simulink model "Robot_DH"  (R2023b)
settings: Solver=VariableStepAuto  StartTime=0.0  StopTime=7  RelTol=1e-3
values from neighbouring files (symbols this model uses):
  a1 = 40    [FK.m]    (also in IK_Analytical.m = 0.04; IK_MDH.m = 0.04; IK_Position.m = 0.04; IK_Solver.m = 0.04)
  a2 = 275    [FK.m]    (also in IK_Analytical.m = 0.275; IK_MDH.m = 0.275; IK_Position.m = 0.275; IK_Solver.m = 0.275)
  a3 = 25    [FK.m]    (also in IK_Analytical.m = 0.025; IK_MDH.m = 0.025; IK_Position.m = 0.025; IK_Solver.m = 0.025)
  d1 = 342    [FK.m]    (also in IK_Analytical.m = 0.342; IK_MDH.m = 0.342; IK_Position.m = 0.342; IK_Solver.m = 0.342)
  d4 = 280    [FK.m]    (also in IK_Analytical.m = 0.28; IK_MDH.m = 0.28; IK_Position.m = 0.28; IK_Solver.m = 0.28)
  DH = @(a,alpha,d,theta) [      cos(theta)            -sin(theta)             0              a ... (first row only)    [FK.m]    (also in set_mode_parameter.m = [)
  dt = 73    [FK.m]    (also in IK_Position.m = 0.073; IK_Solver.m = 0.073; diagnose_IK.m = 0.073; init_robot_arm_system.m = 0.087)
  fc1 = 0    [set_mode_parameter.m]
  fc2 = 0    [set_mode_parameter.m]
  fc3 = 0    [set_mode_parameter.m]
  fc4 = 0    [set_mode_parameter.m]
  fc5 = 0    [set_mode_parameter.m]
  fc6 = 0    [set_mode_parameter.m]
  fv1 = 0    [set_mode_parameter.m]
  fv2 = 0    [set_mode_parameter.m]
  fv3 = 0    [set_mode_parameter.m]
  fv4 = 0    [set_mode_parameter.m]
  fv5 = 0    [set_mode_parameter.m]
  fv6 = 0    [set_mode_parameter.m]
  Ia1 = 0    [set_mode_parameter.m]
  Ia2 = 0    [set_mode_parameter.m]
  Ia3 = 0    [set_mode_parameter.m]
  Ia4 = 0    [set_mode_parameter.m]
  Ia5 = 0    [set_mode_parameter.m]
  Ia6 = 0    [set_mode_parameter.m]
  Ic111 = 0    [set_mode_parameter.m]
  Ic112 = 0    [set_mode_parameter.m]
  Ic113 = 0    [set_mode_parameter.m]
  Ic122 = 0    [set_mode_parameter.m]
  Ic123 = 0    [set_mode_parameter.m]
  Ic133 = 1.3676    [set_mode_parameter.m]
  Ic211 = 8.8194    [set_mode_parameter.m]
  Ic212 = 0    [set_mode_parameter.m]
  Ic213 = 0    [set_mode_parameter.m]
  Ic222 = 6.0549    [set_mode_parameter.m]
  Ic223 = 0    [set_mode_parameter.m]
  Ic233 = 0.9569    [set_mode_parameter.m]
  Ic311 = 0.0332    [set_mode_parameter.m]
  Ic312 = 0    [set_mode_parameter.m]
  Ic313 = 0    [set_mode_parameter.m]
  Ic322 = 1.8442    [set_mode_parameter.m]
  Ic323 = 0    [set_mode_parameter.m]
  Ic333 = 1.0560    (= 1.056)    [set_mode_parameter.m]
  Ic411 = 0.1448    [set_mode_parameter.m]
  Ic412 = 0    [set_mode_parameter.m]
  Ic413 = 0    [set_mode_parameter.m]
  Ic422 = 0.0015    [set_mode_parameter.m]
  Ic423 = 0    [set_mode_parameter.m]
  Ic433 = 0.0822    [set_mode_parameter.m]
  Ic511 = 0    [set_mode_parameter.m]
  Ic512 = 0    [set_mode_parameter.m]
  Ic513 = 0    [set_mode_parameter.m]
  Ic522 = 0.0121    [set_mode_parameter.m]
  Ic523 = 0    [set_mode_parameter.m]
  Ic533 = 0.0299    [set_mode_parameter.m]
  Ic611 = 0.0134    [set_mode_parameter.m]
  Ic612 = 0    [set_mode_parameter.m]
  Ic613 = 0    [set_mode_parameter.m]
  Ic622 = 0    [set_mode_parameter.m]
  Ic623 = 0    [set_mode_parameter.m]
  Ic633 = 0.0051    [set_mode_parameter.m]
  joint_limits = joint_limits_deg    [set_mode_parameter.m]
  m = (c1*px + s1*py) - dt*(c1*ax + s1*ay) - a1    [IK_6DOF_Robot.m]    (also in IK_MDH.m = pwx_1 - a1; IK_MDH_Robot.m = rho - a1)
  m1 = 0.167    [set_mode_parameter.m]
  m2 = 1    [set_mode_parameter.m]
  m3 = 0.5    [set_mode_parameter.m]
  m4 = 0.333    [set_mode_parameter.m]
  m5 = 0.25    [set_mode_parameter.m]
  m6 = 0.2    [set_mode_parameter.m]
  mc11 = 0    [set_mode_parameter.m]
  mc12 = 0    [set_mode_parameter.m]
  mc13 = 0.2    [set_mode_parameter.m]
  mc21 = 0.1291    [set_mode_parameter.m]
  mc22 = 0    [set_mode_parameter.m]
  mc23 = 3.3117    [set_mode_parameter.m]
  mc31 = 1.6484    [set_mode_parameter.m]
  mc32 = 0    [set_mode_parameter.m]
  mc33 = 0.8748    [set_mode_parameter.m]
  mc41 = 0.3200    (= 0.32)    [set_mode_parameter.m]
  mc42 = 0.2324    [set_mode_parameter.m]
  mc43 = 0.7083    [set_mode_parameter.m]
  mc51 = 0.4574    [set_mode_parameter.m]
  mc52 = 0    [set_mode_parameter.m]
  mc53 = 0.6427    [set_mode_parameter.m]
  mc61 = 0.3200    (= 0.32)    [set_mode_parameter.m]
  mc62 = -0.0513    [set_mode_parameter.m]
  mc63 = 0.6417    [set_mode_parameter.m]
  MDH = [ ... (first row only)    [FK_MDH.m]    (also in optimize_MDH_params.m = [x(1:6), [0; 0; 0.275; 0.025; 0; 0],         [0.342; 0.040; ; set_mode_parameter.m; test_222.m)
  N = size(waypoints, 2)    [run_trajectory.m]
  R1 = [0 0 1 ... (first row only)    [set_mode_parameter.m]    (also in test_20251215.m)
  s = zc - d(1)    [inverse_kinematics_6dof.m]
  XB4 = SerialLink([L1 L2 L3 L4 L5 L6], 'name', 'XB4')    [Toolbox_Motheds_1.m]
undefined symbols (not defined in the file or in its folder): X, Y, Z
libraries: sm_lib x56, nesl_utility x31, robotcorelib x2, simulink x2
(part 2 of 2)

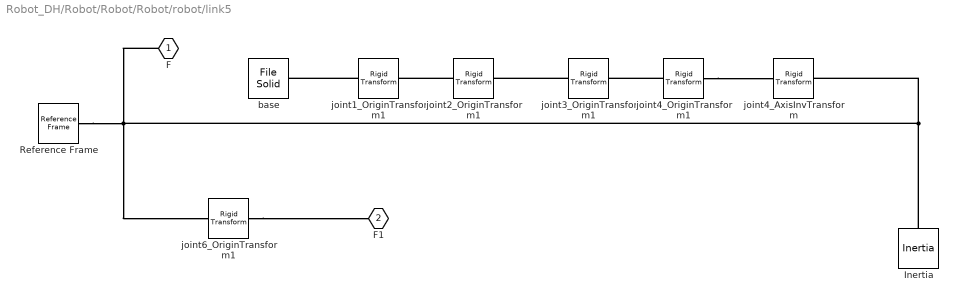
== system Robot_DH/Robot/Robot/Robot/robot/link5 ==
  Inertia : sm_lib/Body Elements/Inertia  InertiaType=Custom  Mass=m5  MassUnits=kg  CenterOfMass=[mc51 mc52 mc53]  CenterOfMassUnits=m  MomentsOfInertia=[Ic511 Ic522 Ic533]  MomentsOfInertiaUnits=kg*m^2  ProductsOfInertia=[Ic523 Ic513 Ic512]  ProductsOfInertiaUnits=kg*m^2  GraphicType=Marker  MarkerShape=Inertia  MarkerSize=20  GraphicVisPropType=SimpleVisualProperties  GraphicDiffuseColor=[0.5 0.5 0.5]  GraphicSpecularColor=[0.5 0.5 0.5 1.0]  GraphicAmbientColor=[0.15 0.15 0.15 1.0]  GraphicEmissiveColor=[0.0 0.0 0.0 1.0]  GraphicShininess=75  GraphicOpacity=1.0
  Reference Frame : sm_lib/Frames and Transforms/Reference Frame
  base : sm_lib/Body Elements/File Solid  ExtGeomFileName=/home/jiehuang/Documents/Custom-Robot/Matlab_Study/Matlab2023Project/IntroductionBook/程序/XB4模型/XB4-5.STL  UnitType=Custom  ExtGeomFileUnits=mm  StepReaderType=HEX  ExportConvexHullGeometry=off  InertiaType=Custom  Mass=0  MassUnits=kg  CenterOfMass=[0 0 0]  CenterOfMassUnits=m  MomentsOfInertia=[0 0 0]  MomentsOfInertiaUnits=kg*m^2  ProductsOfInertia=[0 0 0]  ProductsOfInertiaUnits=kg*m^2  BasedOnType=Density  Density=1000  DensityUnits=kg/(m^3)  DoExposeReferenceFrame=on  SerializedFrames=<Frames/>  GraphicType=FromGeometry  MarkerShape=Sphere  MarkerSize=10  GraphicVisPropType=SimpleVisualProperties  GraphicDiffuseColor=[0.5 0.5 0.5]  GraphicSpecularColor=[0.5 0.5 0.5 1.0]  GraphicAmbientColor=[0.15 0.15 0.15 1.0]  GraphicEmissiveColor=[0.0 0.0 0.0 1.0]  GraphicShininess=75  GraphicOpacity=1.0
  joint1_OriginTransform1 : sm_lib/Frames and Transforms/Rigid Transform  TranslationMethod=Cartesian  TranslationStandardOffset=0  TranslationStandardOffsetUnits=m  TranslationStandardAxis=+Z  TranslationCartesianOffset=[0 0 d1]  TranslationCartesianOffsetUnits=m  TranslationROffset=0  TranslationROffsetUnits=m  TranslationZOffset=0  TranslationZOffsetUnits=m  TranslationThetaOffset=0  TranslationThetaOffsetUnits=deg  RotationMethod=RotationSequence  RotationAngleUnits=deg  RotationStandardAxis=+Z  RotationAngle=0.0  RotationArbitraryAxis=[0 0 1]  FollAlignAxisA=+X  BaseAlignAxisA=+Y  FollAlignAxisB=+Y  BaseAlignAxisB=+Z  RotationSequenceAxes=BaseAxes  RotationSequence=XYZ  RotationSequenceAngles=[0 0 0]  RotationSequenceAnglesUnits=rad  RotationMatrix=[1 0 0; 0 1 0; 0 0 1]  Quaternion=[1 0 0 0]
  joint2_OriginTransform1 : sm_lib/Frames and Transforms/Rigid Transform  TranslationMethod=Cartesian  TranslationStandardOffset=0  TranslationStandardOffsetUnits=m  TranslationStandardAxis=+Z  TranslationCartesianOffset=[a1 0 0]  TranslationCartesianOffsetUnits=m  TranslationROffset=0  TranslationROffsetUnits=m  TranslationZOffset=0  TranslationZOffsetUnits=m  TranslationThetaOffset=0  TranslationThetaOffsetUnits=deg  RotationMethod=RotationSequence  RotationAngleUnits=deg  RotationStandardAxis=+Z  RotationAngle=0.0  RotationArbitraryAxis=[0 0 1]  FollAlignAxisA=+X  BaseAlignAxisA=+Y  FollAlignAxisB=+Y  BaseAlignAxisB=+Z  RotationSequenceAxes=FollowerAxes  RotationSequence=XYZ  RotationSequenceAngles=[-pi/2 0 -pi/2]  RotationSequenceAnglesUnits=rad  RotationMatrix=[1 0 0; 0 1 0; 0 0 1]  Quaternion=[1 0 0 0]
  joint3_OriginTransform1 : sm_lib/Frames and Transforms/Rigid Transform  TranslationMethod=Cartesian  TranslationStandardOffset=0  TranslationStandardOffsetUnits=m  TranslationStandardAxis=+Z  TranslationCartesianOffset=[a2 0 0]  TranslationCartesianOffsetUnits=m  TranslationROffset=0  TranslationROffsetUnits=m  TranslationZOffset=0  TranslationZOffsetUnits=m  TranslationThetaOffset=0  TranslationThetaOffsetUnits=deg  RotationMethod=RotationSequence  RotationAngleUnits=deg  RotationStandardAxis=+Z  RotationAngle=0.0  RotationArbitraryAxis=[0 0 1]  FollAlignAxisA=+X  BaseAlignAxisA=+Y  FollAlignAxisB=+Y  BaseAlignAxisB=+Z  RotationSequenceAxes=FollowerAxes  RotationSequence=XYZ  RotationSequenceAngles=[0 0 0]  RotationSequenceAnglesUnits=rad  RotationMatrix=[1 0 0; 0 1 0; 0 0 1]  Quaternion=[1 0 0 0]
  joint4_AxisInvTransform : sm_lib/Frames and Transforms/Rigid Transform  TranslationMethod=Cartesian  TranslationStandardOffset=0  TranslationStandardOffsetUnits=m  TranslationStandardAxis=+Z  TranslationCartesianOffset=[0 0 0]  TranslationCartesianOffsetUnits=m  TranslationROffset=0  TranslationROffsetUnits=m  TranslationZOffset=0  TranslationZOffsetUnits=m  TranslationThetaOffset=0  TranslationThetaOffsetUnits=deg  RotationMethod=RotationSequence  RotationAngleUnits=rad  RotationStandardAxis=+Z  RotationAngle=1.570796  RotationArbitraryAxis=[0 1 0]  FollAlignAxisA=+X  BaseAlignAxisA=+Y  FollAlignAxisB=+Y  BaseAlignAxisB=+Z  RotationSequenceAxes=FollowerAxes  RotationSequence=XYZ  RotationSequenceAngles=[pi/2 0 0]  RotationSequenceAnglesUnits=rad  RotationMatrix=[1 0 0; 0 1 0; 0 0 1]  Quaternion=[1 0 0 0]
  joint4_OriginTransform1 : sm_lib/Frames and Transforms/Rigid Transform  TranslationMethod=Cartesian  TranslationStandardOffset=0  TranslationStandardOffsetUnits=m  TranslationStandardAxis=+Z  TranslationCartesianOffset=[a3 d4 0]  TranslationCartesianOffsetUnits=m  TranslationROffset=0  TranslationROffsetUnits=m  TranslationZOffset=0  TranslationZOffsetUnits=m  TranslationThetaOffset=0  TranslationThetaOffsetUnits=deg  RotationMethod=RotationSequence  RotationAngleUnits=deg  RotationStandardAxis=+Z  RotationAngle=0.0  RotationArbitraryAxis=[0 0 1]  FollAlignAxisA=+X  BaseAlignAxisA=+Y  FollAlignAxisB=+Y  BaseAlignAxisB=+Z  RotationSequenceAxes=FollowerAxes  RotationSequence=XYZ  RotationSequenceAngles=[-pi/2 0 0]  RotationSequenceAnglesUnits=rad  RotationMatrix=[1 0 0; 0 1 0; 0 0 1]  Quaternion=[1 0 0 0]
  joint6_OriginTransform1 : sm_lib/Frames and Transforms/Rigid Transform  TranslationMethod=Cartesian  TranslationStandardOffset=0  TranslationStandardOffsetUnits=m  TranslationStandardAxis=+Z  TranslationCartesianOffset=[0 0 0]  TranslationCartesianOffsetUnits=m  TranslationROffset=0  TranslationROffsetUnits=m  TranslationZOffset=0  TranslationZOffsetUnits=m  TranslationThetaOffset=0  TranslationThetaOffsetUnits=deg  RotationMethod=RotationSequence  RotationAngleUnits=deg  RotationStandardAxis=+Z  RotationAngle=0.0  RotationArbitraryAxis=[0 0 1]  FollAlignAxisA=+X  BaseAlignAxisA=+Y  FollAlignAxisB=+Y  BaseAlignAxisB=+Z  RotationSequenceAxes=FollowerAxes  RotationSequence=XYZ  RotationSequenceAngles=[-pi/2 0 0]  RotationSequenceAnglesUnits=rad  RotationMatrix=[1 0 0; 0 1 0; 0 0 1]  Quaternion=[1 0 0 0]
  F : PMIOPort  Side=Left
  F1 : PMIOPort  Port=2  Side=Right
  connections:
  Reference Frame/RConn1 -- Inertia/RConn1 -- joint4_AxisInvTransform/RConn1 -- F/RConn1 -- joint6_OriginTransform1/LConn1
  joint6_OriginTransform1/RConn1 -- F1/RConn1
  joint1_OriginTransform1/LConn1 -- base/RConn1
  joint3_OriginTransform1/LConn1 -- joint2_OriginTransform1/RConn1
  joint4_OriginTransform1/LConn1 -- joint3_OriginTransform1/RConn1
  joint2_OriginTransform1/LConn1 -- joint1_OriginTransform1/RConn1
  joint4_OriginTransform1/RConn1 -- joint4_AxisInvTransform/LConn1

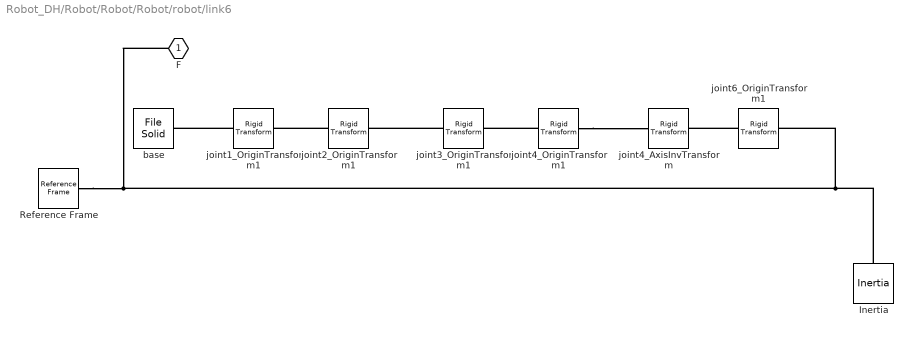
== system Robot_DH/Robot/Robot/Robot/robot/link6 ==
  Inertia : sm_lib/Body Elements/Inertia  InertiaType=Custom  Mass=m6  MassUnits=kg  CenterOfMass=[mc61 mc62 mc63]  CenterOfMassUnits=m  MomentsOfInertia=[Ic611 Ic622 Ic633 ]  MomentsOfInertiaUnits=kg*m^2  ProductsOfInertia=[Ic623 Ic613 Ic612]  ProductsOfInertiaUnits=kg*m^2  GraphicType=Marker  MarkerShape=Inertia  MarkerSize=20  GraphicVisPropType=SimpleVisualProperties  GraphicDiffuseColor=[0.5 0.5 0.5]  GraphicSpecularColor=[0.5 0.5 0.5 1.0]  GraphicAmbientColor=[0.15 0.15 0.15 1.0]  GraphicEmissiveColor=[0.0 0.0 0.0 1.0]  GraphicShininess=75  GraphicOpacity=1.0
  Reference Frame : sm_lib/Frames and Transforms/Reference Frame
  base : sm_lib/Body Elements/File Solid  ExtGeomFileName=/home/jiehuang/Documents/Custom-Robot/Matlab_Study/Matlab2023Project/IntroductionBook/程序/XB4模型/XB4-6.STL  UnitType=Custom  ExtGeomFileUnits=mm  StepReaderType=HEX  ExportConvexHullGeometry=off  InertiaType=Custom  Mass=0  MassUnits=kg  CenterOfMass=[0 0 0]  CenterOfMassUnits=m  MomentsOfInertia=[0 0 0]  MomentsOfInertiaUnits=kg*m^2  ProductsOfInertia=[0 0 0]  ProductsOfInertiaUnits=kg*m^2  BasedOnType=Density  Density=1000  DensityUnits=kg/(m^3)  DoExposeReferenceFrame=on  SerializedFrames=<Frames/>  GraphicType=FromGeometry  MarkerShape=Sphere  MarkerSize=10  GraphicVisPropType=SimpleVisualProperties  GraphicDiffuseColor=[0.5 0.5 0.5]  GraphicSpecularColor=[0.5 0.5 0.5 1.0]  GraphicAmbientColor=[0.15 0.15 0.15 1.0]  GraphicEmissiveColor=[0.0 0.0 0.0 1.0]  GraphicShininess=75  GraphicOpacity=1.0
  joint1_OriginTransform1 : sm_lib/Frames and Transforms/Rigid Transform  TranslationMethod=Cartesian  TranslationStandardOffset=0  TranslationStandardOffsetUnits=m  TranslationStandardAxis=+Z  TranslationCartesianOffset=[0 0 d1]  TranslationCartesianOffsetUnits=m  TranslationROffset=0  TranslationROffsetUnits=m  TranslationZOffset=0  TranslationZOffsetUnits=m  TranslationThetaOffset=0  TranslationThetaOffsetUnits=deg  RotationMethod=RotationSequence  RotationAngleUnits=deg  RotationStandardAxis=+Z  RotationAngle=0.0  RotationArbitraryAxis=[0 0 1]  FollAlignAxisA=+X  BaseAlignAxisA=+Y  FollAlignAxisB=+Y  BaseAlignAxisB=+Z  RotationSequenceAxes=BaseAxes  RotationSequence=XYZ  RotationSequenceAngles=[0 0 0]  RotationSequenceAnglesUnits=rad  RotationMatrix=[1 0 0; 0 1 0; 0 0 1]  Quaternion=[1 0 0 0]
  joint2_OriginTransform1 : sm_lib/Frames and Transforms/Rigid Transform  TranslationMethod=Cartesian  TranslationStandardOffset=0  TranslationStandardOffsetUnits=m  TranslationStandardAxis=+Z  TranslationCartesianOffset=[a1 0 0]  TranslationCartesianOffsetUnits=m  TranslationROffset=0  TranslationROffsetUnits=m  TranslationZOffset=0  TranslationZOffsetUnits=m  TranslationThetaOffset=0  TranslationThetaOffsetUnits=deg  RotationMethod=RotationSequence  RotationAngleUnits=deg  RotationStandardAxis=+Z  RotationAngle=0.0  RotationArbitraryAxis=[0 0 1]  FollAlignAxisA=+X  BaseAlignAxisA=+Y  FollAlignAxisB=+Y  BaseAlignAxisB=+Z  RotationSequenceAxes=FollowerAxes  RotationSequence=XYZ  RotationSequenceAngles=[-pi/2 0 -pi/2]  RotationSequenceAnglesUnits=rad  RotationMatrix=[1 0 0; 0 1 0; 0 0 1]  Quaternion=[1 0 0 0]
  joint3_OriginTransform1 : sm_lib/Frames and Transforms/Rigid Transform  TranslationMethod=Cartesian  TranslationStandardOffset=0  TranslationStandardOffsetUnits=m  TranslationStandardAxis=+Z  TranslationCartesianOffset=[a2 0 0]  TranslationCartesianOffsetUnits=m  TranslationROffset=0  TranslationROffsetUnits=m  TranslationZOffset=0  TranslationZOffsetUnits=m  TranslationThetaOffset=0  TranslationThetaOffsetUnits=deg  RotationMethod=RotationSequence  RotationAngleUnits=deg  RotationStandardAxis=+Z  RotationAngle=0.0  RotationArbitraryAxis=[0 0 1]  FollAlignAxisA=+X  BaseAlignAxisA=+Y  FollAlignAxisB=+Y  BaseAlignAxisB=+Z  RotationSequenceAxes=FollowerAxes  RotationSequence=XYZ  RotationSequenceAngles=[0 0 0]  RotationSequenceAnglesUnits=rad  RotationMatrix=[1 0 0; 0 1 0; 0 0 1]  Quaternion=[1 0 0 0]
  joint4_AxisInvTransform : sm_lib/Frames and Transforms/Rigid Transform  TranslationMethod=Cartesian  TranslationStandardOffset=0  TranslationStandardOffsetUnits=m  TranslationStandardAxis=+Z  TranslationCartesianOffset=[0 0 0]  TranslationCartesianOffsetUnits=m  TranslationROffset=0  TranslationROffsetUnits=m  TranslationZOffset=0  TranslationZOffsetUnits=m  TranslationThetaOffset=0  TranslationThetaOffsetUnits=deg  RotationMethod=RotationSequence  RotationAngleUnits=rad  RotationStandardAxis=+Z  RotationAngle=1.570796  RotationArbitraryAxis=[0 1 0]  FollAlignAxisA=+X  BaseAlignAxisA=+Y  FollAlignAxisB=+Y  BaseAlignAxisB=+Z  RotationSequenceAxes=FollowerAxes  RotationSequence=XYZ  RotationSequenceAngles=[pi/2 0 0]  RotationSequenceAnglesUnits=rad  RotationMatrix=[1 0 0; 0 1 0; 0 0 1]  Quaternion=[1 0 0 0]
  joint4_OriginTransform1 : sm_lib/Frames and Transforms/Rigid Transform  TranslationMethod=Cartesian  TranslationStandardOffset=0  TranslationStandardOffsetUnits=m  TranslationStandardAxis=+Z  TranslationCartesianOffset=[a3 d4 0]  TranslationCartesianOffsetUnits=m  TranslationROffset=0  TranslationROffsetUnits=m  TranslationZOffset=0  TranslationZOffsetUnits=m  TranslationThetaOffset=0  TranslationThetaOffsetUnits=deg  RotationMethod=RotationSequence  RotationAngleUnits=deg  RotationStandardAxis=+Z  RotationAngle=0.0  RotationArbitraryAxis=[0 0 1]  FollAlignAxisA=+X  BaseAlignAxisA=+Y  FollAlignAxisB=+Y  BaseAlignAxisB=+Z  RotationSequenceAxes=FollowerAxes  RotationSequence=XYZ  RotationSequenceAngles=[-pi/2 0 0]  RotationSequenceAnglesUnits=rad  RotationMatrix=[1 0 0; 0 1 0; 0 0 1]  Quaternion=[1 0 0 0]
  joint6_OriginTransform1 : sm_lib/Frames and Transforms/Rigid Transform  TranslationMethod=Cartesian  TranslationStandardOffset=0  TranslationStandardOffsetUnits=m  TranslationStandardAxis=+Z  TranslationCartesianOffset=[0 0 0]  TranslationCartesianOffsetUnits=m  TranslationROffset=0  TranslationROffsetUnits=m  TranslationZOffset=0  TranslationZOffsetUnits=m  TranslationThetaOffset=0  TranslationThetaOffsetUnits=deg  RotationMethod=RotationSequence  RotationAngleUnits=deg  RotationStandardAxis=+Z  RotationAngle=0.0  RotationArbitraryAxis=[0 0 1]  FollAlignAxisA=+X  BaseAlignAxisA=+Y  FollAlignAxisB=+Y  BaseAlignAxisB=+Z  RotationSequenceAxes=FollowerAxes  RotationSequence=XYZ  RotationSequenceAngles=[-pi/2 0 0]  RotationSequenceAnglesUnits=rad  RotationMatrix=[1 0 0; 0 1 0; 0 0 1]  Quaternion=[1 0 0 0]
  F : PMIOPort  Side=Left
  connections:
  Reference Frame/RConn1 -- joint6_OriginTransform1/RConn1 -- Inertia/RConn1 -- F/RConn1
  joint6_OriginTransform1/LConn1 -- joint4_AxisInvTransform/RConn1
  joint1_OriginTransform1/LConn1 -- base/RConn1
  joint3_OriginTransform1/LConn1 -- joint2_OriginTransform1/RConn1
  joint4_OriginTransform1/RConn1 -- joint4_AxisInvTransform/LConn1
  joint4_OriginTransform1/LConn1 -- joint3_OriginTransform1/RConn1
  joint2_OriginTransform1/LConn1 -- joint1_OriginTransform1/RConn1

== matlab function Robot_DH/MATLAB Function ==
  data: p input; R input; T output
function T = BuildT(p, R)
% BuildT  根据固定旋转矩阵 R 和输入位置 p 构建齐次变换矩阵 T
% 输入:
%   p[3x1] - 末端位置向量 [x; y; z]
% 输出:
%   T[4x4] - 齐次变换矩阵

% 固定旋转矩阵 R
% R = [0, 0, 1;
%      0, -1, 0;
%      1, 0, 0];

% 构建齐次矩阵
T = [R, p(:);     % p(:) 确保为列向量
     0 0 0 1];

end

== matlab function Robot_DH/FK/MATLAB Function ==
  data: Radian input; KPS44 output
function KPS44 = FK_DH(Radian)
% FK using Standard DH parameters (替代原MDH)
% 输入:  Radian[1x6] 六个关节角 (rad)
% 输出:  KPS44[4x4] 末端在基坐标系下的齐次变换矩阵 (m)
%
% 零位姿: [0 0 1 0.393; 0 -1 0 0; 1 0 0 0.642; 0 0 0 1]
% 标准DH参数（对应XB4）:
% 关节i: theta_i(输入+偏移) | d_i    | a_i     | alpha_i
%  1    : Radian(1)        | 0.342  | 0.040   | -pi/2
%  2    : Radian(2)-pi/2   | 0      | 0.275   | 0
%  3    : Radian(3)        | 0      | 0.025   | -pi/2
%  4    : Radian(4)        | 0.280  | 0       | pi/2
%  5    : Radian(5)        | 0      | 0       | -pi/2
%  6    : Radian(6)        | 0.073  | 0       | 0

theta = Radian(:);  % 转为列向量

%% 标准DH参数表 (单位: m, rad)
% 每行: [alpha_i, a_i, d_i, theta_offset]
DH = [
    -pi/2,    0.040,    0.342,    0;      % 关节1
     0,       0.275,    0,        -pi/2;      % 关节2 
    -pi/2,    0.025,    0,        0;      % 关节3
     pi/2,    0,        0.280,    0;      % 关节4
    -pi/2,    0,        0,        0;      % 关节5
     0,       0,        0.073,    0;      % 关节6
];

%% 正运动学计算（标准DH）
T = eye(4);  % 初始化为单位矩阵（基坐标系->0号坐标系）

for i = 1:6
    alpha = DH(i,1);  % alpha_i: 绕X_i旋转角度
    a     = DH(i,2);  % a_i: 沿X_i平移距离
    d     = DH(i,3);  % d_i: 沿Z_{i-1}平移距离
    offset= DH(i,4);  % theta_i的偏移量
    
    theta_i = theta(i) + offset;  % 最终关节角（输入+偏移）
    
    % 标准DH变换矩阵公式
    % T_{i-1,i} = Rot(Z_{i-1}, θ_i) * Trans(Z_{i-1}, d_i) * Trans(X_i, a_i) * Rot(X_i, α_i)
    ct = cos(theta_i);
    st = sin(theta_i);
    ca = cos(alpha);
    sa = sin(alpha);
    
    T_i = [ct,   -st*ca,    st*sa,   a*ct;
           st,    ct*ca,   -ct*sa,   a*st;
           0,      sa,       ca,      d;
           0,      0,        0,       1];
    
    T = T * T_i;  % 累积变换（基坐标系->i号坐标系）
end

KPS44 = T;
end

== matlab function Robot_DH/Robot/Robot/Robot/robot/Jm ==
  data: u input; y output; Jm input
function y = fcn(u,Jm)
%#codegen

% Jm=[200; 250; 150; 100; 50; 20];%关节惯性
y = Jm.*u;
end

== matlab function Robot_DH/Robot/Robot/Robot/robot/friction ==
  data: u input; y output; fv input; fc input
function y = fcn(u,fv,fc)
%#codegen


% fv1=100; fc1=80; fv2=150; fc2=100; fv3=100; fc3=50; fv4=80; fc4=80; fv5=50; fc5=30; fv6=30; fc6=10;
fv1=fv(1); fc1=fc(1); fv2=fv(2); fc2=fc(2); fv3=fv(3); fc3=fc(3); fv4=fv(4); fc4=fc(4); fv5=fv(5); fc5=fc(5); fv6=fv(6); fc6=fc(6);
y=[0;0;0;0;0;0];
y(1)=(fv1*u(1)+fc1*sign(u(1)));
y(2)=(fv2*u(2)+fc2*sign(u(2)));
y(3)=(fv3*u(3)+fc3*sign(u(3)));
y(4)=(fv4*u(4)+fc4*sign(u(4)));
y(5)=(fv5*u(5)+fc5*sign(u(5)));
y(6)=(fv6*u(6)+fc6*sign(u(6)));

end

== matlab function Robot_DH/MATLAB Function1 ==
  data: joint_thetas_in input; theta_ret output; thetas output; theta_diffs output; D_H input; best_diff_index output
function [theta_ret, thetas, theta_diffs, best_diff_index] = selectBestSolution_Simple(joint_thetas_in, D_H)
%#codegen
% selectBestSolution_Simple - 选择最优解 (全弧度版本)
%
% 输入: 
%   joint_thetas_in - 6x8 矩阵，8组逆运动学解 (单位: 弧度) [theta1; ...; theta6]
%   D_H             - 6x4 MDH参数矩阵 (单位: 长度m, 角度rad)
%
% 输出:
%   theta_ret       - 6x1 最优解 (单位: 弧度)
%   thetas          - 6x8 所有解 (单位: 弧度)
%   theta_diffs     - 1x8 差异值
%   best_diff_index - 最优解索引

    % 保持维度一致，我们在内部使用 6xN 的形式方便处理，不需要转置成 8x6
    % 输入已经是 6x8 (6个关节，8组解)
    thetas = joint_thetas_in; 
    theta_diffs = zeros(1, 8);
    
    % 持久变量保存当前角度 (6x1 列向量)
    persistent current_theta
    if isempty(current_theta)
        current_theta = zeros(6, 1);
    end
    
    % 遍历8组解
    for k = 1:8
        % 提取第 k 组解 (6x1)
        theta_k = thetas(:, k);
        
        % 计算调整后的角度和差异
        [theta_adj, theta_diff] = joint_theta_change(theta_k, current_theta, D_H);
        
        % 更新解矩阵 (存储调整后的值)
        thetas(:, k) = theta_adj;
        theta_diffs(k) = theta_diff;
    end
    
    % 选择差异最小的解
    [~, best_diff_index] = min(theta_diffs);
    theta_ret = thetas(:, best_diff_index); % 返回 6x1
    
    % 更新当前位置
    current_theta = theta_ret;
end

function [theta_out, theta_diff] = joint_theta_change(theta_in, current_theta, D_H)
    % 输入输出均为 6x1 列向量，单位全为弧度
    theta_out = zeros(6, 1);
    theta_diff = 0;
    
    for i = 1:6
        % 1. 处理输入角度 (归一化到 0 ~ 2pi)
        tmp_theta = mod(theta_in(i), 2*pi);
        if tmp_theta < 0
             tmp_theta = tmp_theta + 2*pi;
        end
        
        % 2. 处理初始偏移 (D_H(i,4) 是 theta 偏移，单位为弧度)
        % 注意：如果您前面的 IK 算法算出的已经是关节角 theta，
        % 这里可能不需要再减去 D_H(i,4)。
        % 如果您的机械臂零位不是数学零位，则需要这行；否则建议直接 init_theta = 0。
        % 此处为了通过编译，保留逻辑但确保全是弧度。
        init_theta = mod(D_H(i, 4), 2*pi); 
        
        % 计算相对角度
        val = tmp_theta - init_theta;
        
        % 3. 归一化到 [-pi, pi] (即 -180 ~ 180 度)
        % 这是为了让机器人走最短路径
        val = mod(val + pi, 2*pi) - pi;
        
        theta_out(i) = val;
        
        % 4. 计算差异 (加权)
        % 权重: 关节1最大(7-1=6), 关节6最小(7-6=1)
        diff_val = abs(theta_out(i) - current_theta(i));
        
        % 处理跨越 2pi 的差异 (例如 -3.14 和 3.14 实际上很近)
        if diff_val > pi
            diff_val = 2*pi - diff_val;
        end
        
        theta_diff = theta_diff + (7 - i) * diff_val;
    end
end

== matlab function Robot_DH/MATLAB Function2 ==
  data: T input; q_sols output; a1 input; a2 input; a3 input; d1 input; d4 input; d6 input
function q_sols = IK_DH_All_Sols(T, a1, a2, a3, d1, d4, d6)
% IK_DH_All_Sols 计算6自由度机器人的逆运动学的所有8组解
%
% 输入:
%   T:    [4x4] 目标末端齐次变换矩阵
%   a1:   关节1的连杆长度 (DH参数a1)
%   a2:   关节2的连杆长度 (DH参数a2)
%   a3:   关节3的连杆长度 (DH参数a3)
%   d1:   关节1的连杆偏距 (DH参数d1)
%   d4:   关节4的连杆偏距 (DH参数d4)
%   d6:   关节6的连杆偏距 (DH参数d6，末端执行器长度)
%
% 输出:
%   q_sols: [6x8] 矩阵。每一列代表一组解 [th1; th2; ...; th6]
%           如果某组解不可达（超出工作空间），该列填充 NaN。

    % === 1. 几何参数预计算 ===
    L2 = a2;
    L3 = sqrt(a3^2 + d4^2); % 连杆3等效长度
    phi = atan2(d4, a3);    % 连杆3弯曲角

    % === 2. 腕心位置计算 (Position) ===
    % 从末端 T 回推到腕心 (Wrist Center)
    nx = T(1,1); ny = T(2,1); nz = T(3,1);
    ox = T(1,2); oy = T(2,2); oz = T(3,2);
    ax = T(1,3); ay = T(2,3); az = T(3,3);
    px = T(1,4); py = T(2,4); pz = T(3,4);

    xc = px - d6 * ax;
    yc = py - d6 * ay;
    zc = pz - d6 * az;

    % === 3. 循环计算8组解 ===
    % 初始化输出矩阵 (6行 x 8列)
    q_sols = nan(6, 8);
    col_idx = 1;

    % 循环 1: 肩部 (Shoulder) - 前方/后方
    % conf_arm = 1 (Front), -1 (Back)
    for conf_arm = [1, -1]
        
        % 计算 Theta 1
        % 计算基础角度
        theta1_base = atan2(yc, xc);
        if conf_arm == -1
            theta1 = theta1_base + pi;
        else
            theta1 = theta1_base;
        end
        % 归一化到 (-pi, pi]
        theta1 = atan2(sin(theta1), cos(theta1));

        % 定义旋转后的平面坐标 (Planar Coordinates)
        xy_mag = sqrt(xc^2 + yc^2);
        
        if conf_arm == 1
            % 前方: 腕心在 a1 前方
            x_in = xy_mag - a1;
        else
            % 后方: 腕心在 a1 "后方"
            x_in = -xy_mag - a1; 
        end
        
        z_in = zc - d1;

        % 循环 2: 肘部 (Elbow) - 上/下
        % conf_elbow = 1 (Up), -1 (Down)
        for conf_elbow = [1, -1]
            
            % 使用余弦定理计算 Theta 3
            dist_sq = x_in^2 + z_in^2;
            cos_th3_star = (dist_sq - L2^2 - L3^2) / (2 * L2 * L3);

            % 检查是否超出工作空间
            if abs(cos_th3_star) > 1
                % 该分支无解，跳过（保持 NaN）
                col_idx = col_idx + 2; % 跳过两个 Wrist 解
                continue; 
            end
            
            sin_th3_star = conf_elbow * sqrt(1 - cos_th3_star^2);
            theta3_star = atan2(sin_th3_star, cos_th3_star);
            
            theta3 = theta3_star + phi;

            % 计算 Theta 2
            % beta 是三角形内角
            beta = atan2(L3 * sin(theta3_star), L2 + L3 * cos(theta3_star));
            % psi 是腕心向量角度
            psi = atan2(z_in, x_in);
            
            theta2 = psi - beta;

            % === 4. 腕部姿态计算 (Orientation) ===
            % 计算前三轴的旋转矩阵 R0_3
            
            % R0_1 (alpha = -pi/2)
            c1 = cos(theta1); s1 = sin(theta1);
            R0_1 = [c1, 0, -s1; s1, 0, c1; 0, -1, 0];
            
            % R1_2 (alpha = 0)
            c2 = cos(theta2); s2 = sin(theta2);
            R1_2 = [c2, -s2, 0; s2, c2, 0; 0, 0, 1];
            
            % R2_3 (alpha = -pi/2)
            c3 = cos(theta3); s3 = sin(theta3);
            R2_3 = [c3, 0, -s3; s3, 0, c3; 0, -1, 0];
            
            R0_3 = R0_1 * R1_2 * R2_3;
            
            % 计算腕部所需的局部旋转 R3_6
            % R3_6 = (R0_3)^T * R_goal
            R_goal = T(1:3, 1:3);
            R3_6 = R0_3' * R_goal;
            
            r13 = R3_6(1,3); r23 = R3_6(2,3);
            r31 = R3_6(3,1); r32 = R3_6(3,2); r33 = R3_6(3,3);

            % 循环 3: 腕部 (Wrist) - 翻转/不翻转
            % conf_wrist = 1 (No Flip), -1 (Flip)
            for conf_wrist = [1, -1]
                
                % 计算 Theta 5
                th5_sin = sqrt(r31^2 + r32^2);
                
                if conf_wrist == -1
                    th5_sin = -th5_sin;
                end
                
                theta5 = atan2(th5_sin, r33);

                % 计算 Theta 4 和 Theta 6
                if abs(th5_sin) < 1e-4
                    % 奇异点: Theta 5 接近 0，万向节死锁
                    theta4 = 0; % 任意指定
                    theta6 = atan2(R3_6(2,1), R3_6(1,1)) - theta4;
                else
                    % 正常情况
                    theta4 = atan2(-r23, -r13);
                    theta6 = atan2(-r32, r31);
                end

                % 保存结果到当前列
                q_sols(:, col_idx) = [theta1; theta2; theta3; theta4; theta5; theta6];
                col_idx = col_idx + 1;
            end
        end
    end
end
